simulink model "IMP_LQR_KALMAN_EXPERIMENT"  (R2017b)
settings: Solver=ode1  StartTime=0.0  StopTime=20  FixedStep=0.002  RelTol=1e-3  EnableMultiTasking=on
PreLoadFcn:
  | quanser_aero_lqr
values from neighbouring files (symbols this model uses):
  A_aug = [A B*Cref; zeros(4,4) Aref]    [IMP_LQR_Design.m]
  B_aug = [B; zeros(4,2)]    [IMP_LQR_Design.m]
  C_aug = [C zeros(2,4)]    [IMP_LQR_Design.m]
  J = J'    [IMP_LQR_Design.m]    (also in LQR_Design.m = place(A',C', polesj)'; design.m = place(A',C', polesj)')
  K = [K Cref]    [IMP_LQR_Design.m]    (also in design.m = place(A,B, polesk); quanser_aero_lqr.m = lqr(A,B,Q,R))
  N = K(1:2,1:2)    [IMP_LQR_Design.m]
libraries: simulink_extras x4, quanser_aero x1, quarc_library x1
settings Model: SimulationMode=external  ExtModeTrigDuration=15000  Creator=MLevis  LastModifiedBy=craigr1
settings SolverCC: PositivePriorityOrder=on
settings DataIOCC: LimitDataPoints=on  SaveFormat=Array
settings OptimizationCC: LifeSpan=inf
settings DebuggingCC: SolverPrmCheckMsg=warning  SFUnexpectedBacktrackingDiag=warning  SFNoUnconditionalDefaultTransitionDiag=warning  SFExecutionAtInitializationDiag=none
settings HardwareCC: ProdBitPerPointer=32  ProdBitPerSizeT=32  ProdBitPerPtrDiffT=32  ProdLargestAtomicFloat=None  ProdIntDivRoundTo=Undefined  ProdEndianess=Unspecified  ProdWordSize=32  ProdHWDeviceType=32-bit Generic
settings ModelReferenceCC: PropagateSignalLabelsOutOfModel=off
settings RTWCC: SystemTargetFile=quarc_win64.tlc  TemplateMakefile=quarc_default_tmf  Description=QUARC Win64 Target
settings CodeAppCC: StateflowObjectComments=on
settings STFCustomTargetCC: TargetPreCompLibLocation=C:\PROGRA~3\QUARC\lib\2017b\win64\release  ConcurrentExecutionCompliant=on  GeneratePreprocessorConditionals=Disable all  SystemTargetFile=quarc_win64.tlc
settings GRTTargetCC: TargetPreCompLibLocation=C:\PROGRA~3\QUARC\lib\2017b\win64\release  TargetLangStandard=C89/C90 (ANSI)  ParMdlRefBuildCompliant=off  CompOptLevelCompliant=off  GeneratePreprocessorConditionals=Disable all  CombineOutputUpdateFcns=off  MatFileLogging=off  CPPClassGenCompliant=off  GRTInterface=on  UseToolchainInfoCompliant=off  ExtMode=on  ExtModeMexFile=quarc_comm
settings ConfigComp: CovMetricSettings=dw  CovHtmlReporting=on  CovSaveCumulativeToWorkspaceVar=on  CovSaveSingleToWorkspaceVar=on  CovExternalEMLEnable=off  CovSFcnEnable=off

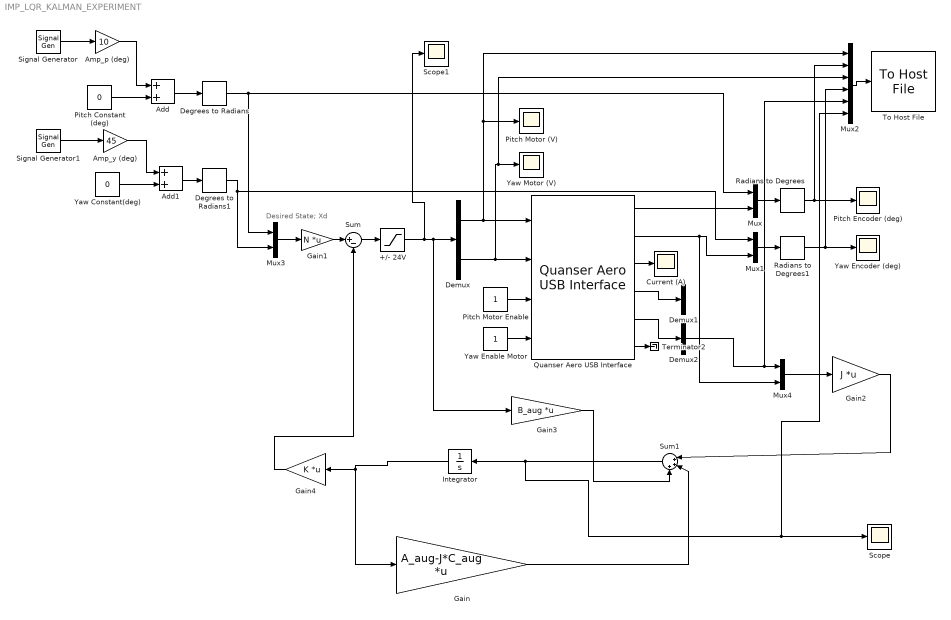
== system IMP_LQR_KALMAN_EXPERIMENT ==
  note: Desired State; Xd
  +/- 24V : Saturate  UpperLimit=24  LowerLimit=-24
  Add : Sum
  Add1 : Sum
  Amp_p (deg) : Gain  Gain=10
  Amp_y (deg) : Gain  Gain=45
  Current (A) : Scope
  Degrees to Radians : simulink_extras/Transformations/Degrees to Radians
  Degrees to Radians1 : simulink_extras/Transformations/Degrees to Radians
  Demux : Demux  Outputs=2
  Demux1 : Demux  Outputs=2
  Demux2 : Demux  Outputs=3
  Gain : Gain  Gain=A_aug-J*C_aug  Multiplication=Matrix(K*u)
  Gain1 : Gain  Gain=N  Multiplication=Matrix(K*u)
  Gain2 : Gain  Gain=J  Multiplication=Matrix(K*u)
  Gain3 : Gain  Gain=B_aug  Multiplication=Matrix(K*u)
  Gain4 : Gain  Gain=K  Multiplication=Matrix(K*u)
  Integrator : Integrator
  Mux{,1,3..4} (4 alike) : Mux  Inputs=2
  Mux2 : Mux  Inputs=6
  Pitch Constant (deg) : Constant  Value=0
  Pitch Encoder (deg) : Scope
  Pitch Motor (V) : Scope
  Pitch Motor Enable : Constant
  Quanser Aero USB Interface : quanser_aero/Quanser Aero USB Interface
  Radians to Degrees : simulink_extras/Transformations/Radians to Degrees
  Radians to Degrees1 : simulink_extras/Transformations/Radians to Degrees
  Scope : Scope
  Scope1 : Scope
  Signal Generator : SignalGenerator  Frequency=1/5
  Signal Generator1 : SignalGenerator  Frequency=1/10
  Sum : Sum  Inputs=|+-
  Sum1 : Sum  Inputs=|+++
  Terminator2 : Terminator
  To Host File : quarc_library/Sinks/To Host/To Host File  file_name=aero_lqr_rsp23.mat  variable_name=lqr_rsp  decimation=1  sample_time=-1  file_format=MAT-file v.4  options=No header or footer  append=off  final_file_name=aero_lqr_rsp23.mat  bitrate=2000000
  Yaw Constant(deg) : Constant  Value=0
  Yaw Enable Motor : Constant
  Yaw Encoder (deg) : Scope
  Yaw Motor (V) : Scope
  wires:
  Degrees to Radians/1 -> Mux3/1, Mux/1
  Degrees to Radians1/1 -> Mux3/2, Mux1/1
  Signal Generator/1 -> Amp_p (deg)/1
  Pitch Constant (deg)/1 -> Add/2
  Add/1 -> Degrees to Radians/1
  Yaw Constant(deg)/1 -> Add1/2
  Amp_p (deg)/1 -> Add/1
  Signal Generator1/1 -> Amp_y (deg)/1
  Amp_y (deg)/1 -> Add1/1
  Add1/1 -> Degrees to Radians1/1
  Mux/1 -> Radians to Degrees/1
  Radians to Degrees/1 -> Mux2/2, Pitch Encoder (deg)/1
  Radians to Degrees1/1 -> Yaw Encoder (deg)/1, Mux2/4
  Pitch Motor Enable/1 -> Quanser Aero USB Interface/3
  Yaw Enable Motor/1 -> Quanser Aero USB Interface/4
  Sum/1 -> +/- 24V/1
  Demux/1 -> Quanser Aero USB Interface/1, Mux2/1, Pitch Motor (V)/1
  Demux/2 -> Quanser Aero USB Interface/2, Mux2/3, Yaw Motor (V)/1
  Mux1/1 -> Radians to Degrees1/1
  +/- 24V/1 -> Scope1/1, Gain3/1, Demux/1
  Quanser Aero USB Interface/3 -> Current (A)/1
  Quanser Aero USB Interface/2 -> Mux4/2, Mux1/2
  Quanser Aero USB Interface/6 -> Terminator2/1
  Mux2/1 -> To Host File/1
  Quanser Aero USB Interface/4 -> Demux1/1
  Mux3/1 -> Gain1/1
  Gain1/1 -> Sum/1
  Gain2/1 -> Sum1/1
  Mux4/1 -> Gain2/1
  Quanser Aero USB Interface/1 -> Mux/2
  Gain/1 -> Sum1/2
  Sum1/1 -> Mux2/6, Scope/1, Integrator/1
  Gain3/1 -> Sum1/3
  Integrator/1 -> Gain/1, Gain4/1
  Gain4/1 -> Sum/2
  Quanser Aero USB Interface/5 -> Demux2/1
  Demux2/2 -> Mux2/5, Mux4/1
